simulink model "GPR_MPC_CARSIM"  (Simulink 10.1)
settings: Solver=ode45  StartTime=0.0  StopTime=200  FixedStep=0.01  RelTol=1e-3  EnableMultiTasking=on
libraries: Solver_SF x1
settings Model: Creator=xuwei
settings DataIOCC: LimitDataPoints=on  SignalLoggingSaveFormat=ModelDataLogs
settings OptimizationCC: ExpressionDepthLimit=2147483647
settings DebuggingCC: SolverPrmCheckMsg=warning  FcnCallInpInsideContextMsg=warning  StateNameClashWarn=warning

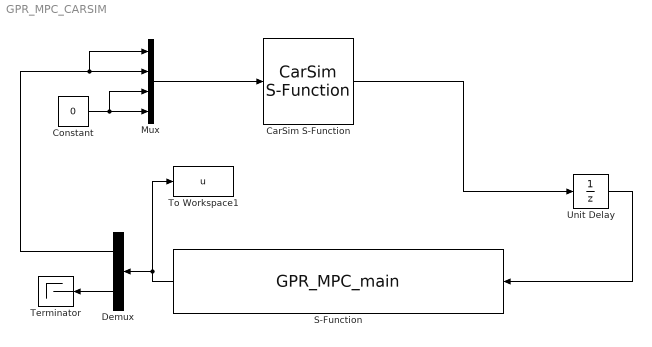
== system GPR_MPC_CARSIM ==
  CarSim S-Function : Solver_SF/CarSim S-Function  Priority=1  SIMFILE=simfile.sim  Run_RTs=off  vs_state_ind=Run  StopMode_ind=Vehicle Model
  Constant : Constant  Value=0
  Demux : Demux  Outputs=[1 9]
  Mux : Mux
  S-Function : S-Function  FunctionName=GPR_MPC_main  SFunctionDeploymentMode=off  EnableBusSupport=off
  Terminator : Terminator
  To Workspace1 : ToWorkspace  VariableName=u  SaveFormat=Structure  SampleTime=-1
  Unit Delay : UnitDelay  SampleTime=-1  HasFrameUpgradeWarning=on
  wires:
  S-Function/1 -> Demux/1, To Workspace1/1
  Demux/2 -> Terminator/1
  Mux/1 -> CarSim S-Function/1
  Demux/1 -> Mux/2, Mux/1
  Constant/1 -> Mux/3, Mux/4
  Unit Delay/1 -> S-Function/1
  CarSim S-Function/1 -> Unit Delay/1
